simulink model "host_udp_demo"  (Simulink 7.3)
settings: Solver=VariableStepDiscrete  StartTime=0.0  StopTime=inf  RelTol=1e-3
settings Model: Creator=Krisada  LastModifiedBy=Krisada

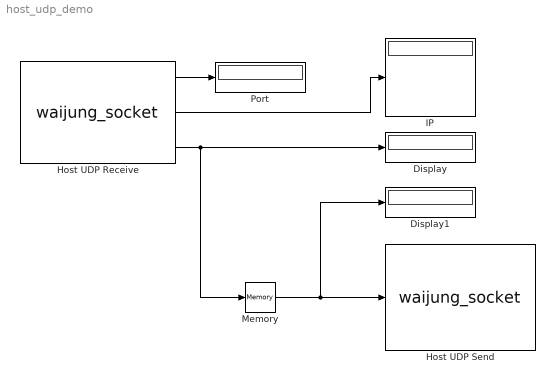
== system host_udp_demo ==
  Display : Display
  Display1 : Display
  Host UDP Receive : S-Function  Priority=1  FunctionName=waijung_socket  Parameters=conf,inputporttype,inputportwidth,outputporttype,outputportwidth,address,port,optionstring,sampletime,blockid,options  EnableBusSupport=off  mask(waijung_socket){conf=HostReceive, protocol=UDP, port=7, netadapter=Intel(R) 82579LM Gigabit Network Connection, address=192.168.1.10, echo=off, transfer=Blocking, timeout=5, datasource=Ports, datatype=uint8, datacount=2, porttype_double=0, porttype_single=0, porttype_int8=0, porttype_uint8=0, porttype_int16=0, porttype_uint16=0, porttype_int32=0, porttype_uint32=1, portpinstr=0, sampletime=0.001, blockid=HostUDPReceive, inputporttype=[], inputportwidth=[], inputportlabel={}, outputporttype=[5,3,7], outputportwidth=[1,4,], outputportlabel={'Remote Port','Remote IP(1:4)','uint32 D0'}, compat=0, optionstring=["UDP","7","192","168","1","21","Non-blocking","PortData","uint8_t","2","Send","off"], options=[7,2,1,5000,0]}
      mask prompts: conf "Configuration"; netadapter "Host Network Adapter"; echo "Echo (Return the receiving data back to sender)"; timeout "Timeout (Seconds)"; datasource "Data"; datatype "Data type"; datacount "Port width"; porttype_double "Number of data port, type DOUBLE"; porttype_single "Number of data port, type SINGLE"; porttype_int8 "Number of data port, type INT8"; porttype_uint8 "Number of data port, type UINT8"; porttype_int16 "Number of data port, type INT16"; porttype_uint16 "Number of data port, type UINT16"; porttype_int32 "Number of data port, type INT32"; porttype_uint32 "Number of data port, type UINT32"; portpinstr "Port Pin String"; sampletime "Sample time (sec)"; blockid "Block ID"; inputporttype "Input Port Type"; inputportwidth "Input Port Width"; inputportlabel "Input Port Label"; outputporttype "Output Port Type"; outputportwidth "Output Port Width"; outputportlabel "Output port label"; compat "Compatibility (Reserved for future use)"; optionstring "String(s) to be passed to TLC"; options "Sim options"
      mask help:
      | Port:
      |  - Port number to open for data receive.
      | Transfer:
      |  - Blocking: CPU is blocked durring wait for data.
      | Timeout:
      |  - Timeout in seconds for wait for data.
      mask init:
      | waijung_socket_callback('init');
      mask Help: web(fullfile(waijungdocroot,'waijung_socket_host_udp_receive.htm'), '-browser')
      mask StyleString: popup(HostSend|HostReceive|TargetSend|TargetReceive),popup(TCP|UDP),edit,popup(Intel(R) 82579LM Gigabit Network Connection),edit,checkbox,popup(Blocking|Non-blocking),edit,popup(Ports|Vector|BufferStream),popup(double|single|int8|uint8|int16|uint16|int32|uint32),edit,edit,edit,edit,edit,edit,edit,edit,edit,edit,edit,edit,edit,edit,edit,edit,edit,edit,edit,edit,edit
      mask CallbackString: waijung_socket_callback('conf');|||waijung_socket_callback('netadapter');|||||waijung_socket_callback('datasource');|||waijung_socket_callback('datatype');|waijung_socket_callback('datatype');|waijung_socket_callback('datatype');|waijung_socket_callback('datatype');|waijung_socket_callback('datatype');|waijung_socket_callback('datatype');|waijung_socket_callback('datatype');|waijung_socket_callback('datatype');||waijung_socket_callback('sampletime');|waijung_socket_callback('blockid');|||||||||
      mask Display: text(0.05, 0.5, '[Host UDP Receive]\nPort: 7\nTs (sec): 0.001','ver','middle','hor','left'); port_label('output', 1,'Remote Port'); port_label('output', 2,'Remote IP(1:4)'); port_label('output', 3,'uint32 D0');
  Host UDP Send : S-Function  Priority=0  FunctionName=waijung_socket  Parameters=conf,inputporttype,inputportwidth,outputporttype,outputportwidth,address,port,optionstring,sampletime,blockid,options  EnableBusSupport=off  mask(waijung_socket){conf=HostSend, protocol=UDP, variableipport=off, netadapter=Intel(R) 82579LM Gigabit Network Connection, blockid=192.168.1.10, port=7, address=192.168.1.31, echo=off, transfer=Blocking, timeout=5, datasource=Ports, datatype=uint8, datacount=2, porttype_double=0, porttype_single=0, porttype_int8=0, porttype_uint8=0, porttype_int16=0, porttype_uint16=0, porttype_int32=0, porttype_uint32=1, portpinstr=0, sampletime=inf, inputporttype=[7], inputportwidth=[1], inputportlabel={'D0 uint32'}, outputporttype=[], outputportwidth=[], outputportlabel={}, compat=0, optionstring=["UDP","7","192","168","1","21","Non-blocking","PortData","uint8_t","2","Send","off"], options=[7,2,0,5000,0]}
      mask prompts: conf "Configuration"; variableipport "Variable Destination IP/Port"; netadapter "Host Network Adapter"; blockid "Address"; port "Destination port"; address "Destination address"; echo "Echo (Return the receiving data back to sender)"; timeout "Timeout (Seconds)"; datasource "Data"; datatype "Data type"; datacount "Port width"; porttype_double "Number of data port, type DOUBLE"; porttype_single "Number of data port, type SINGLE"; porttype_int8 "Number of data port, type INT8"; porttype_uint8 "Number of data port, type UINT8"; porttype_int16 "Number of data port, type INT16"; porttype_uint16 "Number of data port, type UINT16"; porttype_int32 "Number of data port, type INT32"; porttype_uint32 "Number of data port, type UINT32"; portpinstr "Port Pin String"; sampletime "Sample time (sec)"; inputporttype "Input Port Type"; inputportwidth "Input Port Width"; inputportlabel "Input Port Label"; outputporttype "Output Port Type"; outputportwidth "Output Port Width"; outputportlabel "Output port label"; compat "Compatibility (Reserved for future use)"; optionstring "String(s) to be passed to TLC"; options "Sim options"
      mask help:
      | Destintion port:
      |  - Specify port number to send data packet to.
      | Destination address:
      |  - IP address of destination.
      | Transfer:
      |  Blocking: CPU is blocked during data sending.
      |  Non-Blocking: Not support for Host UDP send.
      mask init:
      | waijung_socket_callback('init');
      mask Help: web(fullfile(waijungdocroot,'waijung_socket_host_udp_send.htm'), '-browser')
      mask StyleString: popup(HostSend|HostReceive|TargetSend|TargetReceive),popup(TCP|UDP),checkbox,popup(Intel(R) 82579LM Gigabit Network Connection),edit,edit,edit,checkbox,popup(Blocking|Non-blocking),edit,popup(Ports|Vector),popup(double|single|int8|uint8|int16|uint16|int32|uint32),edit,edit,edit,edit,edit,edit,edit,edit,edit,edit,edit,edit,edit,edit,edit,edit,edit,edit,edit,edit
      mask CallbackString: waijung_socket_callback('conf');||waijung_socket_callback('conf');||waijung_socket_callback('blockid');||||||waijung_socket_callback('datasource');|||waijung_socket_callback('datatype');|waijung_socket_callback('datatype');|waijung_socket_callback('datatype');|waijung_socket_callback('datatype');|waijung_socket_callback('datatype');|waijung_socket_callback('datatype');|waijung_socket_callback('datatype');|waijung_socket_callback('datatype');||waijung_socket_callback('sampletime');|||||||||
      mask Display: text(0.95, 0.5, '[Host UDP Send]\nAddr: 192.168.1.31\nPort: 7\nTs (sec): 0.001','ver','middle','hor','right'); port_label('input', 1,'D0 uint32');
  IP : Display
      settings: Format=decimal (Stored Integer)
  Memory : Memory  InheritSampleTime=on
  Port : Display
  wires:
  Host UDP Receive/3 -> Display/1, Memory/1
  Memory/1 -> Host UDP Send/1, Display1/1
  Host UDP Receive/1 -> Port/1
  Host UDP Receive/2 -> IP/1
